simulink model "guideLines1"  (R2016b)
settings: Solver=ode45  StartTime=0.0  StopTime=10.0  RelTol=1e-3  EnableMultiTasking=on
libraries: sampleLib x2
settings Model: Creator=ktrinh  LastModifiedBy=hbourbou
settings OptimizationCC: LifeSpan=inf
settings DebuggingCC: SFUnexpectedBacktrackingDiag=warning  SFNoUnconditionalDefaultTransitionDiag=warning  SFExecutionAtInitializationDiag=none
settings HardwareCC: ProdBitPerSizeT=32  ProdBitPerPtrDiffT=32  ProdWordSize=32  ProdHWDeviceType=Specified
settings GRTTargetCC: TargetLangStandard=C89/C90 (ANSI)  GeneratePreprocessorConditionals=Disable all
settings ConfigComp: CovMetricSettings=dw  CovHtmlReporting=on  CovSaveCumulativeToWorkspaceVar=on  CovSaveSingleToWorkspaceVar=on  CovExternalEMLEnable=off

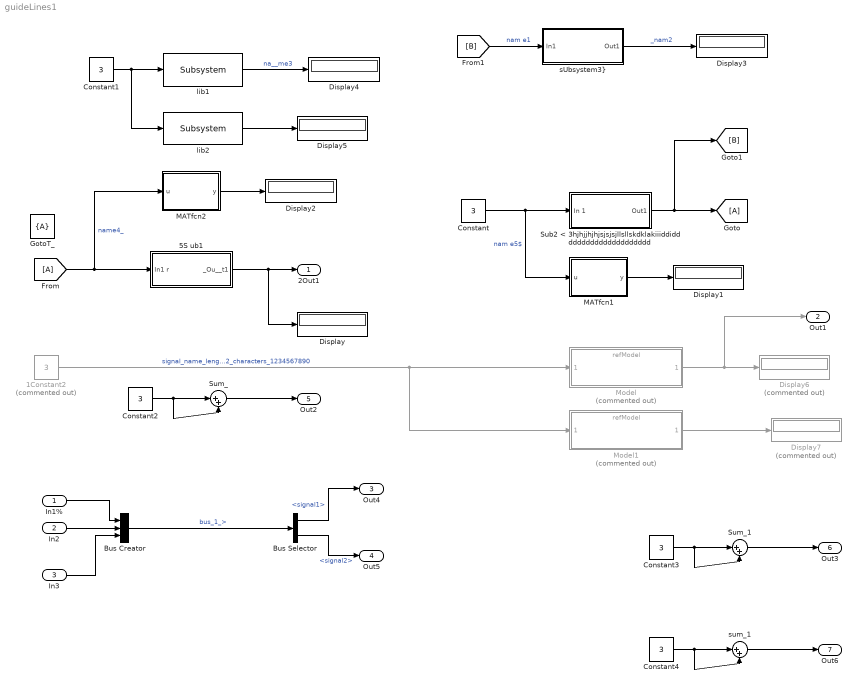
== system guideLines1 ==
  In1% : Inport  OutDataTypeStr=double  PortDimensions=1
  In2 : Inport  Port=2  OutDataTypeStr=double  PortDimensions=1
  In3 : Inport  Port=3  OutDataTypeStr=double  PortDimensions=1
  1Constant2 : Constant  Commented=on  Value=3
  5S ub1 : Subsystem
      settings: AttributesFormatString=%<NamePlacement>
  Bus Creator : BusCreator  Inputs=3
  Bus Selector : BusSelector  OutputSignals=signal1,signal2
  Constant{,1..4} (5 alike) : Constant  Value=3
  Display{,1..5} (6 alike) : Display
  Display6 : Display  Commented=on
  Display7 : Display  Commented=on
  GotoT_ : GotoTagVisibility
  MATfcn1 : MATLAB Function  TreatAsAtomicUnit=on
  MATfcn2 : MATLAB Function  TreatAsAtomicUnit=on
  Model : ModelReference  Commented=on  ModelNameDialog=refModel.slx  SimulationMode=Normal  ModelReferenceVersion=1.49
  Model1 : ModelReference  Commented=on  ModelNameDialog=refModel.slx  SimulationMode=Normal  ModelReferenceVersion=1.49
  Sub2 < 3hjhjjhjhjsjsjsjllsllskdklakiiiddiddddddddddddddddddddd : Subsystem
  Sum_ : Sum  Inputs=|++
  Sum_1 : Sum  Inputs=|++
  lib1 : sampleLib/Subsystem
  lib2 : sampleLib/Subsystem
  "sUbsystem3}" : Subsystem
  sum_1 : Sum  Inputs=|++
  2Out1 : Outport
  Out1 : Outport  Port=2
  Out4 : Outport  Port=3
  Out5 : Outport  Port=4
  Out2 : Outport  Port=5
  Out3 : Outport  Port=6
  Out6 : Outport  Port=7
  wires:
  5S ub1/1(_Ou__t1) -> Display/1, 2Out1/1
  Sub2 < 3hjhjjhjhjsjsjsjllsllskdklakiiiddiddddddddddddddddddddd/1(Out1) -> [B], [A]
  Constant/1 -> MATfcn1/1(u), Sub2 < 3hjhjjhjhjsjsjsjllsllskdklakiiiddiddddddddddddddddddddd/1(In 1)  "nam e5$"
  MATfcn1/1(y) -> Display1/1
  [A] -> MATfcn2/1(u), 5S ub1/1(In1 r)  "name4_"
  MATfcn2/1(y) -> Display2/1
  [B] -> "sUbsystem3}"/1(In1)  "nam e1"
  "sUbsystem3}"/1(Out1) -> Display3/1  "_nam2"
  lib1/1 -> Display4/1  "na__me3"
  Constant1/1 -> lib2/1, lib1/1
  lib2/1 -> Display5/1
  1Constant2/1 -> Model/1, Model1/1  "signal_name_length_longer_than_32_characters_1234567890"
  Model/1 -> Out1/1, Display6/1
  Model1/1 -> Display7/1
  In2/1 -> Bus Creator/2
  In3/1 -> Bus Creator/3
  In1%/1 -> Bus Creator/1
  Bus Selector/1 -> Out4/1  "<signal1>"
  Bus Creator/1 -> Bus Selector/1  "bus_1_>"
  Bus Selector/2 -> Out5/1  "<signal2>"
  Constant2/1 -> Sum_/2, Sum_/1
  Sum_/1 -> Out2/1
  Sum_1/1 -> Out3/1
  Constant3/1 -> Sum_1/2, Sum_1/1
  sum_1/1 -> Out6/1
  Constant4/1 -> sum_1/2, sum_1/1

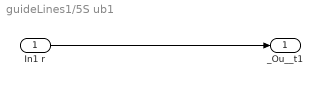
== system guideLines1/5S ub1 ==
  In1 r : Inport
  _Ou__t1 : Outport
  wires:
  In1 r/1 -> _Ou__t1/1

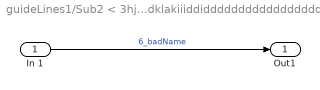
== system guideLines1/Sub2 < 3hjhjjhjhjsjsjsjllsllskdklakiiiddiddddddddddddddddddddd ==
  In 1 : Inport
  Out1 : Outport
  wires:
  In 1/1 -> Out1/1  "6_badName"

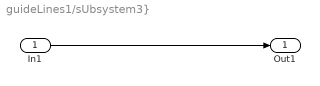
== system guideLines1/sUbsystem3} ==
  In1 : Inport
  Out1 : Outport
  wires:
  In1/1 -> Out1/1

== matlab function guideLines1/MATfcn2 ==
  data: u input; y output
function y = fcn(u)
%#codegen

y = u+2;

== matlab function guideLines1/MATfcn1 ==
  data: u input; y output
function y = fcn(u)
%#codegen

y = u+2;
